simulink model "req12"  (R2019a)
settings: Solver=FixedStepAuto  StartTime=0.0  StopTime=100  RelTol=1e-3
settings Model: Creator=e40014285  LastModifiedBy=e40014285
settings ConfigComp: CovEnable=on  CovScope=ReferencedModels  RecordCoverage=on  CovHTMLOptions=-sRT=1 -sVT=0 -aTS=1 -bRG=1 -bTC=1 -hTR=0 -nFC=0 -nFD=1 -scm=1 -bcm=1 -xEv=0 -xEM=0  CovHtmlReporting=on  CovCumulativeReport=on  DVModelCoverageObjectives=EnhancedMCDC  DVTestSuiteOptimization=Auto  DVDetectOutOfBounds=on  DVReportPDFFormat=on  DVRebuildModelRepresentation=Always

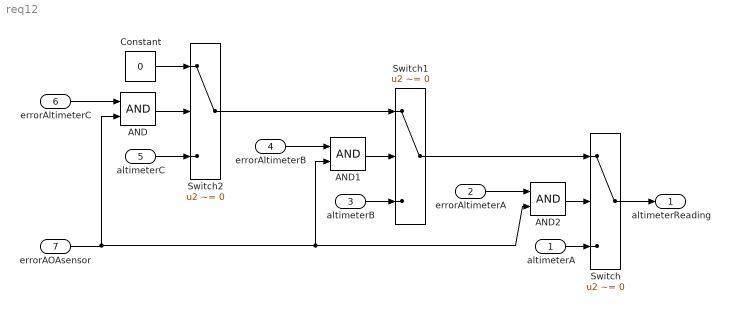
== system req12 ==
  altimeterA : Inport
  errorAltimeterA : Inport  Port=2  OutDataTypeStr=boolean
  altimeterB : Inport  Port=3
  errorAltimeterB : Inport  Port=4  OutDataTypeStr=boolean
  altimeterC : Inport  Port=5
  errorAltimeterC : Inport  Port=6  OutDataTypeStr=boolean
  errorAOAsensor : Inport  Port=7  OutDataTypeStr=boolean
  AND : Logic  AllPortsSameDT=off  OutDataTypeStr=boolean
  AND1 : Logic  AllPortsSameDT=off  OutDataTypeStr=boolean
  AND2 : Logic  AllPortsSameDT=off  OutDataTypeStr=boolean
  Constant : Constant  Value=0
  Switch : Switch  Criteria=u2 ~= 0
  Switch1 : Switch  Criteria=u2 ~= 0
  Switch2 : Switch  Criteria=u2 ~= 0
  altimeterReading : Outport
  wires:
  Switch/1 -> altimeterReading/1
  errorAltimeterA/1 -> AND2/1
  altimeterA/1 -> Switch/3
  Switch1/1 -> Switch/1
  altimeterB/1 -> Switch1/3
  errorAltimeterB/1 -> AND1/1
  errorAltimeterC/1 -> AND/1
  altimeterC/1 -> Switch2/3
  Switch2/1 -> Switch1/1
  Constant/1 -> Switch2/1
  errorAOAsensor/1 -> AND2/2, AND1/2, AND/2
  AND/1 -> Switch2/2
  AND1/1 -> Switch1/2
  AND2/1 -> Switch/2
